simulink model "CSE_STEPRESPONSE_BLOCKDIAGRAM_NO3_CASTOR"  (R2024a)
settings: Solver=VariableStepAuto  StartTime=0.0  StopTime=20  RelTol=1e-3
values from neighbouring files (symbols this model uses):
  G_den3 = [M3 B3 k3]    [CSE_STEPRESPONSE_CODE_NO3_CASTOR.m]    (also in CSE_STEPRESPONSE_CODE_NO3_NO4_CASTOR.m)
  G_num3 = [1]    [CSE_STEPRESPONSE_CODE_NO3_CASTOR.m]    (also in CSE_STEPRESPONSE_CODE_NO3_NO4_CASTOR.m)
settings Model: Creator=Vince Joseph Castor  LastModifiedBy=Vince Joseph Castor

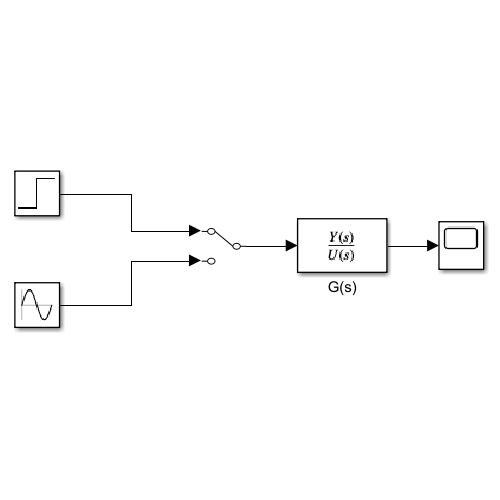
[thumbnail: Simulink's stored preview of the top-level diagram]
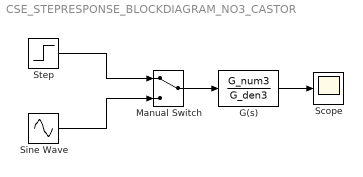
== system CSE_STEPRESPONSE_BLOCKDIAGRAM_NO3_CASTOR ==
  G(s) : TransferFcn  Numerator=G_num3  Denominator=G_den3
  Manual Switch : ManualSwitch
  Scope : Scope
  Sine Wave : Sin  SampleTime=0
  Step : Step  Time=0  SampleTime=0
  wires:
  Step/1 -> Manual Switch/1
  G(s)/1 -> Scope/1
  Manual Switch/1 -> G(s)/1
  Sine Wave/1 -> Manual Switch/2
